simulink model "op_loop_error"  (R2016b)
settings: Solver=VariableStepAuto  StartTime=0.0  StopTime=20  RelTol=1e-3
undefined symbols (not defined in the file or in its folder): A_long, B_long, C_long
libraries: dspsrcs4 x3
settings Model: Creator=yashm  LastModifiedBy=yashm

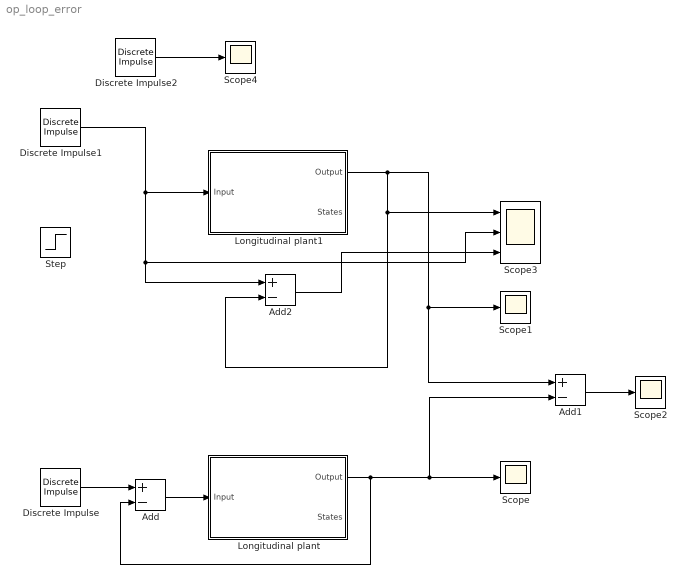
== system op_loop_error ==
  Add : Sum  Inputs=+-
  Add1 : Sum  Inputs=+-
  Add2 : Sum  Inputs=+-
  Discrete Impulse : dspsrcs4/Discrete  Impulse  Delay=0  SampleTime=1  FrameSample=1  OutputFrames=off  dataType=double  isSigned=on  wordLen=16  udDataType=sfix(16)  fracBitsMode=Best precision  numFracBits=15  OutDataTypeStr=double  LastOutDataTypeStr=double
  Discrete Impulse1 : dspsrcs4/Discrete  Impulse  Delay=1  SampleTime=1  FrameSample=1  OutputFrames=off  dataType=double  isSigned=on  wordLen=16  udDataType=sfix(16)  fracBitsMode=Best precision  numFracBits=15  OutDataTypeStr=double  LastOutDataTypeStr=double
  Discrete Impulse2 : dspsrcs4/Discrete  Impulse  Delay=2  SampleTime=1  FrameSample=1  OutputFrames=off  dataType=double  isSigned=on  wordLen=16  udDataType=sfix(16)  fracBitsMode=Best precision  numFracBits=15  OutDataTypeStr=double  LastOutDataTypeStr=double
  Longitudinal plant : Subsystem
  Longitudinal plant1 : Subsystem
  Scope{,1..2,4} (4 alike) : Scope
  Scope3 : Scope  NumInputPorts=3
  Step : Step  SampleTime=0
  wires:
  Longitudinal plant/1(Output) -> Add/2, Add1/2, Scope/1
  Discrete Impulse/1 -> Add/1
  Add/1 -> Longitudinal plant/1(Input)
  Longitudinal plant1/1(Output) -> Scope3/1, Add2/2, Add1/1, Scope1/1
  Add1/1 -> Scope2/1
  Add2/1 -> Scope3/3
  Discrete Impulse1/1 -> Longitudinal plant1/1(Input), Scope3/2, Add2/1
  Discrete Impulse2/1 -> Scope4/1

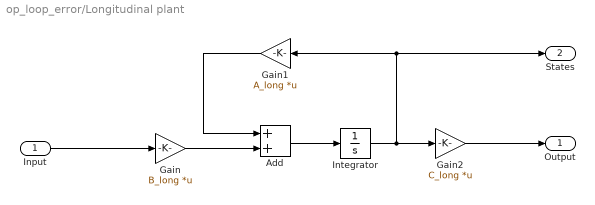
== system op_loop_error/Longitudinal plant ==
  Input : Inport
  Add : Sum
  Gain : Gain  Gain=B_long  Multiplication=Matrix(K*u)
  Gain1 : Gain  Gain=A_long  Multiplication=Matrix(K*u)
  Gain2 : Gain  Gain=C_long  Multiplication=Matrix(K*u)
  Integrator : Integrator
  Output : Outport
  States : Outport  Port=2
  wires:
  Gain2/1 -> Output/1
  Input/1 -> Gain/1
  Gain/1 -> Add/2
  Integrator/1 -> Gain1/1, States/1, Gain2/1
  Add/1 -> Integrator/1
  Gain1/1 -> Add/1

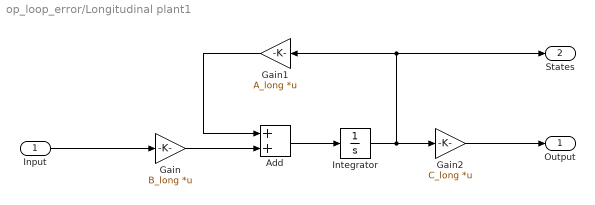
== system op_loop_error/Longitudinal plant1 ==
  Input : Inport
  Add : Sum
  Gain : Gain  Gain=B_long  Multiplication=Matrix(K*u)
  Gain1 : Gain  Gain=A_long  Multiplication=Matrix(K*u)
  Gain2 : Gain  Gain=C_long  Multiplication=Matrix(K*u)
  Integrator : Integrator
  Output : Outport
  States : Outport  Port=2
  wires:
  Gain1/1 -> Add/1
  Add/1 -> Integrator/1
  Integrator/1 -> Gain2/1, States/1, Gain1/1
  Gain/1 -> Add/2
  Input/1 -> Gain/1
  Gain2/1 -> Output/1
